simulink model "n_metro_discret"  (Simulink 7.2)
settings: Solver=ode45  StartTime=0.0  StopTime=L  RelTol=1e-6
undefined symbols (not defined in the file): Amax, Delta, DiscIntNeverNeededParam, K, Ka, Ki, Kv, L, N, Tau, tda, tdd, Te, tpsm
settings Model: Creator=acco  LastModifiedBy=acco
settings DataIOCC: SignalLoggingName=sigsOut
settings DebuggingCC: SaveWithParameterizedLinksMsg=none  SignalResolutionControl=TryResolveAllWithWarning  SolverPrmCheckMsg=none  MultiTaskDSMMsg=warning  MultiTaskCondExecSysMsg=none  StrictBusMsg=None
settings HardwareCC: TargetUnknown=on
settings RTWCC: IncludeERTFirstTime=on

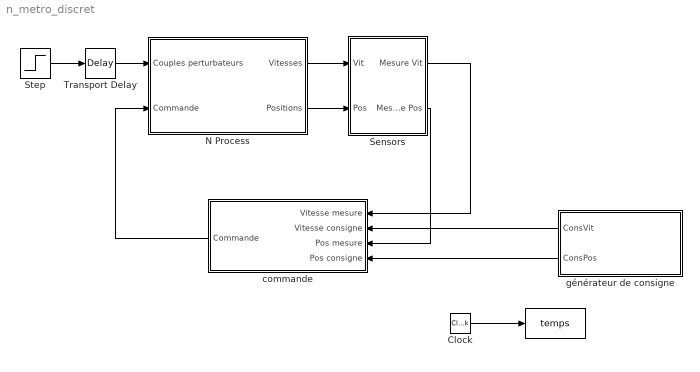
== system n_metro_discret ==
  " " : ToWorkspace  VariableName=temps  SampleTime=Te  SaveFormat=Array
  Clock : DigitalClock  SampleTime=Te
  N Process : Subsystem
  Sensors : Subsystem
  Step : Step  Time=L*0.1  Before=ones(N,1)*0  After=-ones(N,1)*0
  Transport Delay : TransportDelay  DelayTime=N-(1:N)
  commande : Subsystem  Orientation=left  TreatAsAtomicUnit=on
      settings: RTWSystemCode=Function  RTWFcnNameOpts=Use subsystem name  RTWFileNameOpts=Use subsystem name
  générateur de consigne : Subsystem  Orientation=left
  wires:
  Step/1 -> Transport Delay/1
  Clock/1 -> " "/1
  commande/1(Commande) -> N Process/2(Commande)
  générateur de consigne/2(ConsPos) -> commande/4(Pos consigne)
  Transport Delay/1 -> N Process/1(Couples perturbateurs)
  générateur de consigne/1(ConsVit) -> commande/2(Vitesse consigne)
  N Process/1(Vitesses) -> Sensors/1(Vit)
  Sensors/1(Mesure Vit) -> commande/1(Vitesse mesure)
  N Process/2(Positions) -> Sensors/2(Pos)
  Sensors/2(Mesure Pos) -> commande/3(Pos mesure)

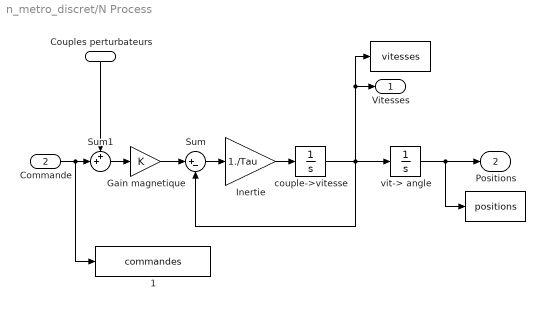
== system n_metro_discret/N Process ==
  Couples perturbateurs : Inport  Orientation=down  OutDataType=sfix(16)  OutScaling=2^0
  Commande : Inport  Port=2  OutDataType=sfix(16)  OutScaling=2^0
  " " : ToWorkspace  VariableName=vitesses  SampleTime=Te  SaveFormat=Array
  "  " : ToWorkspace  VariableName=positions  SampleTime=Te  SaveFormat=Array
  "   1" : ToWorkspace  VariableName=commandes  SampleTime=Te  SaveFormat=Array
  Gain magnetique : Gain  Gain=K  ParameterDataType=sfix(16)  ParameterScaling=2^0  OutDataType=sfix(16)  OutScaling=2^0  SaturateOnIntegerOverflow=on  OutDataTypeStr=Inherit: Same as input  ParamDataTypeStr=Inherit: Same as input
  Inertie : Gain  Gain=1./Tau  ParameterDataType=sfix(16)  ParameterScaling=2^0  OutDataType=sfix(16)  OutScaling=2^0  SaturateOnIntegerOverflow=on  OutDataTypeStr=Inherit: Same as input  ParamDataTypeStr=Inherit: Same as input
  Sum : Sum  Inputs=|+-  OutDataType=sfix(16)  OutScaling=2^0  SaturateOnIntegerOverflow=on
  Sum1 : Sum  Inputs=++|  OutDataType=sfix(16)  OutScaling=2^0  SaturateOnIntegerOverflow=on
  couple->vitesse : Integrator  InitialCondition=zeros(N,1)
  vit-> angle : Integrator  InitialCondition=(0:N-1)*Delta
  Vitesses : Outport  OutDataType=sfix(16)  OutScaling=2^0
  Positions : Outport  Port=2  OutDataType=sfix(16)  OutScaling=2^0
  wires:
  vit-> angle/1 -> "  "/1, Positions/1
  Commande/1 -> "   1"/1, Sum1/2
  Inertie/1 -> couple->vitesse/1
  Gain magnetique/1 -> Sum/1
  Sum/1 -> Inertie/1
  couple->vitesse/1 -> vit-> angle/1, Vitesses/1, " "/1, Sum/2
  Sum1/1 -> Gain magnetique/1
  Couples perturbateurs/1 -> Sum1/1

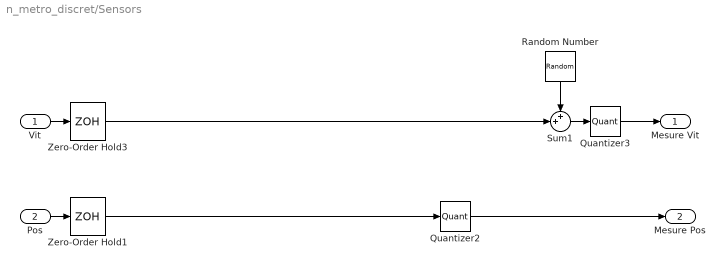
== system n_metro_discret/Sensors ==
  Vit : Inport
  Pos : Inport  Port=2
  Quantizer2 : Quantizer  QuantizationInterval=1
  Quantizer3 : Quantizer  QuantizationInterval=1
  Random Number : RandomNumber  Orientation=down  Mean=zeros(N,1)  Variance=ones(N,1)*50  Seed=rand(N,1)  SampleTime=Te
  Sum1 : Sum  Inputs=++|  OutDataType=sfix(16)  OutScaling=2^0  SaturateOnIntegerOverflow=on
  Zero-Order Hold1 : ZeroOrderHold  SampleTime=Te
  Zero-Order Hold3 : ZeroOrderHold  SampleTime=Te
  Mesure Vit : Outport
  Mesure Pos : Outport  Port=2
  wires:
  Random Number/1 -> Sum1/1
  Vit/1 -> Zero-Order Hold3/1
  Sum1/1 -> Quantizer3/1
  Zero-Order Hold1/1 -> Quantizer2/1
  Quantizer2/1 -> Mesure Pos/1
  Pos/1 -> Zero-Order Hold1/1
  Quantizer3/1 -> Mesure Vit/1
  Zero-Order Hold3/1 -> Sum1/2

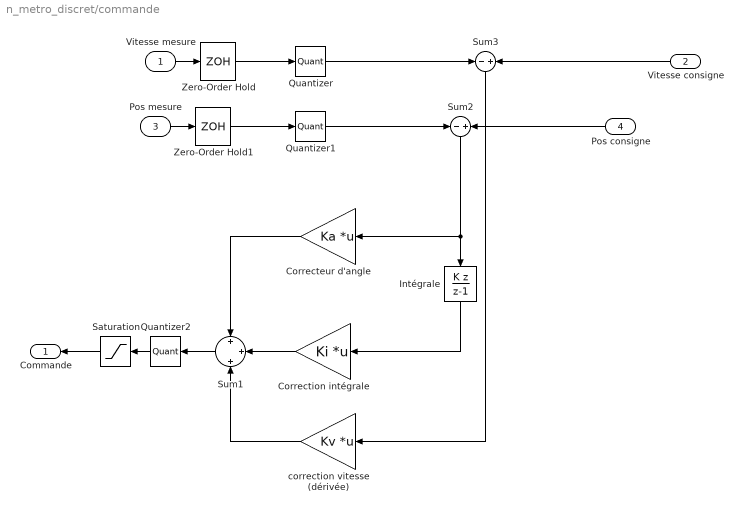
== system n_metro_discret/commande ==
  Vitesse mesure : Inport  OutDataType=sfix(16)  OutScaling=2^0
  Vitesse consigne : Inport  Orientation=left  Port=2  OutDataType=sfix(16)  OutScaling=2^0
  Pos mesure : Inport  Port=3  OutDataType=sfix(16)  OutScaling=2^0
  Pos consigne : Inport  Orientation=left  Port=4  OutDataType=sfix(16)  OutScaling=2^0
  Correcteur d'angle : Gain  Orientation=left  Gain=Ka  Multiplication=Matrix(K*u)  ParameterDataType=sfix(16)  ParameterScaling=2^0  OutDataType=sfix(16)  OutScaling=2^0  SaturateOnIntegerOverflow=on  OutDataTypeStr=Inherit: Same as input  ParamDataTypeStr=Inherit: Same as input
  Correction intégrale : Gain  Orientation=left  Gain=Ki  Multiplication=Matrix(K*u)  ParameterDataType=sfix(16)  ParameterScaling=2^0  OutDataType=sfix(16)  OutScaling=2^0  SaturateOnIntegerOverflow=on  OutDataTypeStr=Inherit: Same as input  ParamDataTypeStr=Inherit: Same as input
  Intégrale : DiscreteIntegrator  Orientation=down  IntegratorMethod=Accumulation: Backward Euler  gainval=1.0*ones(N,1)  InitialCondition=zeros(N,1)  SampleTime=Te  LimitOutput=on  UpperSaturationLimit=4095/max(max(Ki))*ones(N,1)  LowerSaturationLimit=-4095/max(max(Ki))*ones(N,1)  ICPrevOutput=DiscIntNeverNeededParam  ICPrevScaledInput=DiscIntNeverNeededParam
  Quantizer : Quantizer  QuantizationInterval=1
  Quantizer1 : Quantizer  QuantizationInterval=1
  Quantizer2 : Quantizer  Orientation=left  QuantizationInterval=1
  Saturation : Saturate  Orientation=left  UpperLimit=4095  LowerLimit=-4095  OutDataType=sfix(16)  OutScaling=2^0
  Sum1 : Sum  Orientation=left  Inputs=+|+|+  OutDataType=sfix(16)  OutScaling=2^0  SaturateOnIntegerOverflow=on
  Sum2 : Sum  Orientation=down  Inputs=-|+  OutDataType=sfix(16)  OutScaling=2^0  SaturateOnIntegerOverflow=on
  Sum3 : Sum  Orientation=down  Inputs=-|+  OutDataType=sfix(16)  OutScaling=2^0  SaturateOnIntegerOverflow=on
  Zero-Order Hold : ZeroOrderHold  SampleTime=Te
  Zero-Order Hold1 : ZeroOrderHold  SampleTime=Te
  correction vitesse (dérivée) : Gain  Orientation=left  Gain=Kv  Multiplication=Matrix(K*u)  ParameterDataType=sfix(16)  ParameterScaling=2^0  OutDataType=sfix(16)  OutScaling=2^0  SaturateOnIntegerOverflow=on  OutDataTypeStr=Inherit: Same as input  ParamDataTypeStr=Inherit: Same as input
  Commande : Outport  Orientation=left
  wires:
  Sum2/1 -> Intégrale/1, Correcteur d'angle/1
  Correcteur d'angle/1 -> Sum1/1
  Sum3/1 -> correction vitesse (dérivée)/1
  Intégrale/1 -> Correction intégrale/1
  correction vitesse (dérivée)/1 -> Sum1/3
  Correction intégrale/1 -> Sum1/2
  Vitesse consigne/1 -> Sum3/2
  Pos consigne/1 -> Sum2/2
  Vitesse mesure/1 -> Zero-Order Hold/1
  Pos mesure/1 -> Zero-Order Hold1/1
  Sum1/1 -> Quantizer2/1
  Zero-Order Hold/1 -> Quantizer/1
  Zero-Order Hold1/1 -> Quantizer1/1
  Saturation/1 -> Commande/1
  Quantizer/1 -> Sum3/1
  Quantizer1/1 -> Sum2/1
  Quantizer2/1 -> Saturation/1

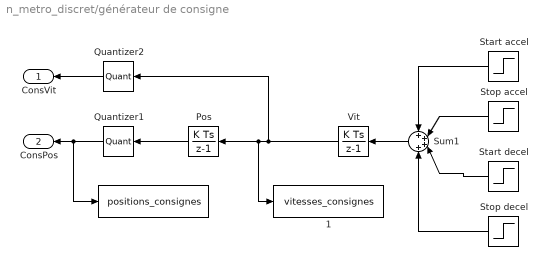
== system n_metro_discret/générateur de consigne ==
  "  " : ToWorkspace  VariableName=positions_consignes  SampleTime=Te  SaveFormat=Array
  "  1" : ToWorkspace  VariableName=vitesses_consignes  SampleTime=Te  SaveFormat=Array
  Pos : DiscreteIntegrator  Orientation=left  InitialCondition=[0:N-1]'*Delta  SampleTime=Te  ICPrevOutput=DiscIntNeverNeededParam  ICPrevScaledInput=DiscIntNeverNeededParam
  Quantizer1 : Quantizer  Orientation=left  QuantizationInterval=1
  Quantizer2 : Quantizer  Orientation=left  QuantizationInterval=1
  Start accel : Step  Orientation=left  Time=tda  Before=ones(N,1)*0  After=ones(N,1)*Amax  SampleTime=Te
  Start decel : Step  Orientation=left  Time=tdd  Before=ones(N,1)*0  After=-ones(N,1)*Amax  SampleTime=Te
  Stop accel : Step  Orientation=left  Time=tda+tpsm  Before=ones(N,1)*0  After=-ones(N,1)*Amax  SampleTime=Te
  Stop decel : Step  Orientation=left  Time=tdd+tpsm  Before=ones(N,1)*0  After=ones(N,1)*Amax  SampleTime=Te
  Sum1 : Sum  Orientation=left  Inputs=++++  OutDataType=sfix(16)  OutScaling=2^0  SaturateOnIntegerOverflow=on
  Vit : DiscreteIntegrator  Orientation=left  InitialCondition=ones(N,1)*0  SampleTime=Te  ICPrevOutput=DiscIntNeverNeededParam  ICPrevScaledInput=DiscIntNeverNeededParam
  ConsVit : Outport  Orientation=left
  ConsPos : Outport  Orientation=left  Port=2
  wires:
  Vit/1 -> Quantizer2/1, Pos/1, "  1"/1
  Pos/1 -> Quantizer1/1
  Start accel/1 -> Sum1/1
  Stop accel/1 -> Sum1/2
  Start decel/1 -> Sum1/3
  Stop decel/1 -> Sum1/4
  Sum1/1 -> Vit/1
  Quantizer2/1 -> ConsVit/1
  Quantizer1/1 -> "  "/1, ConsPos/1
